simulink model "plant_block_swing"  (R2013a)
settings: Solver=ode1  StartTime=0.0  StopTime=120  RelTol=1e-3
undefined symbols (not defined in the file or in its folder): magnitude
libraries: simulink x2
settings Model: SimulationMode=external  ExtModeTrigDuration=50000  Creator=Dro  LastModifiedBy=s4358046
settings DataIOCC: LimitDataPoints=off  SignalLoggingSaveFormat=ModelDataLogs  SignalLoggingName=sigsOut
settings OptimizationCC: ExpressionDepthLimit=2147483647  InitFltsAndDblsToZero=on
settings DebuggingCC: SaveWithParameterizedLinksMsg=none  SignalResolutionControl=TryResolveAllWithWarning  SolverPrmCheckMsg=none  MultiTaskDSMMsg=warning  MultiTaskCondExecSysMsg=none  FcnCallInpInsideContextMsg=UseLocalSettings  StrictBusMsg=None
settings RTWCC: SystemTargetFile=rtwin.tlc  TemplateMakefile=rtwin.tmf  Description=Real-Time Windows Target  ProcessScript=rtwin_make_rtw_hook  IncludeERTFirstTime=on
settings RTWinTargetCC: TargetFcnLib=ansi_tfl_tmw.mat  TargetLibSuffix=_rtwin.lib  TargetPreCompLibLocation=C:\Program Files\MATLAB\R2013a\toolbox\rtw\targets\rtwin\lib\win64  CodeReplacementLibrary=ANSI_C  ModelReferenceCompliant=off  CompOptLevelCompliant=off  RTWinDir=C:/PROGRA~1/MATLAB/R2013a/toolbox/rtw/targets/rtwin  TargetArch=win64

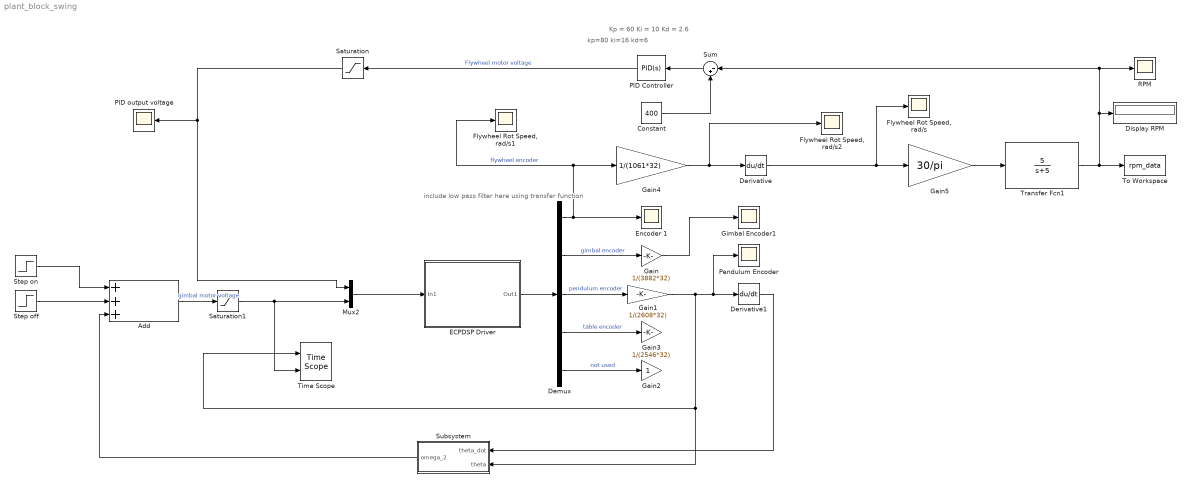
== system plant_block_swing ==
  note: Kp = 60
      | Ki = 10
      | Kd = 2.6
  note: include low pass filter here
      | using transfer function
  note: kp=80
      | ki=16
      | kd=6
  Add : Sum  Inputs=+++
  Constant : Constant  Value=400
  Demux : Demux  Outputs=5
  Derivative : Derivative
  Derivative1 : Derivative
  Display RPM : Display
  ECPDSP Driver : Subsystem  mask{BaseAddr='0xC000', STime=0.008, TimeOutPer=500, HWAccess=on}
      mask prompts: BaseAddr "Base I/O Address"; STime "Sample Time (Sec)"; TimeOutPer "Timeout Period (500 ~ 2000)"; HWAccess "Hardware Access"
      mask Display: color('black');disp('ECPDSP Driver\n upto\n 4 Encs(ADC Channels)\n and 2 Dacs')
  Encoder 1 : Scope
      settings: YMin=1.5e+06  YMax=8.5e+06  SaveName=ScopeData3
  "Flywheel Rot Speed, rad/s" : Scope
  "Flywheel Rot Speed, rad/s1" : Scope
      settings: SaveName=ScopeData2
  "Flywheel Rot Speed, rad/s2" : Scope
      settings: SaveName=ScopeData4
  Gain : Gain  Gain=1/(3882*32)
  Gain1 : Gain  Gain=1/(2608*32)
  Gain2 : Gain
  Gain3 : Gain  Gain=1/(2546*32)
  Gain4 : Gain  Gain=1/(1061*32)
  Gain5 : Gain  Gain=30/pi
  Gimbal Encoder1 : Scope
      settings: YMin=-0.25  YMax=3.25  SaveName=ScopeData9
  Mux2 : Mux  Inputs=2
  PID Controller : simulink/Continuous/PID Controller  Controller=PID  TimeDomain=Continuous-time  SampleTime=1  IntegratorMethod=Forward Euler  FilterMethod=Forward Euler  Form=Parallel  P=60  I=10  D=2.6  N=100  InitialConditionSource=internal  InitialConditionForIntegrator=0  InitialConditionForFilter=0  ExternalReset=none  LimitOutput=off  UpperSaturationLimit=inf  LowerSaturationLimit=-inf  LinearizeAsGain=on  AntiWindupMode=none  Kb=1  TrackingMode=off  Kt=1  PParamMin=[]  PParamMax=[]  IParamMin=[]  IParamMax=[]  DParamMin=[]  DParamMax=[]  NParamMin=[]  NParamMax=[]  KbParamMin=[]  KbParamMax=[]  KtParamMin=[]  KtParamMax=[]  POutMin=[]  POutMax=[]  IOutMin=[]  IOutMax=[]  DOutMin=[]  DOutMax=[]  NOutMin=[]  NOutMax=[]  KbOutMin=[]  KbOutMax=[]  KtOutMin=[]  KtOutMax=[]  IntegratorOutMin=[]  IntegratorOutMax=[]  FilterOutMin=[]  FilterOutMax=[]  SumOutMin=[]  SumOutMax=[]  SumI1OutMin=[]  SumI1OutMax=[]  SumI2OutMin=[]  SumI2OutMax=[]  SumI3OutMin=[]  SumI3OutMax=[]  SumDOutMin=[]  SumDOutMax=[]  SaturationOutMin=[]  SaturationOutMax=[]  IntegratorContinuousStateAttributes=''  IntegratorStateMustResolveToSignalObject=off  IntegratorRTWStateStorageClass=Auto  FilterContinuousStateAttributes=''  FilterStateMustResolveToSignalObject=off  FilterRTWStateStorageClass=Auto
  PID output voltage : Scope
      settings: YMin=400  YMax=421  SaveName=ScopeData6
  Pendulum Encoder : Scope
      settings: YMin=-0.25  YMax=3.25  SaveName=ScopeData5
  RPM : Scope
      settings: YMin=400  YMax=421
  Saturation : Saturate  UpperLimit=32000  LowerLimit=-32000
  Saturation1 : Saturate  UpperLimit=22000  LowerLimit=-22000
  Step off : Step  Time=30.15  After=-14000  SampleTime=0
  Step on : Step  Time=30  After=14000  SampleTime=0
  Subsystem : Subsystem
  Sum : Sum  Inputs=|-+
  Time Scope : TimeScope  NumInputPorts=2  DefaultConfigurationName=spbscopes.TimeScopeBlockCfg
      settings: CopyFcn=scopeextensions.ScopeBlock.callback(gcbh, 'onBlockCopy', gcbh);  DeleteFcn=scopeextensions.ScopeBlock.callback(gcbh, 'onBlockDelete');  PreSaveFcn=scopeextensions.ScopeBlock.callback(gcbh, 'onModelSave');  NameChangeFcn=scopeextensions.ScopeBlock.callback(gcbh, 'onBlockRename');  CloseFcn=scopeextensions.ScopeBlock.callback(gcbh, 'onBlockClose');  PreDeleteFcn=scopeextensions.ScopeBlock.callback(gcbh, 'onBlockPreDelete');
  To Workspace : ToWorkspace  VariableName=rpm_data  SampleTime=-1  SaveFormat=Timeseries
  Transfer Fcn1 : TransferFcn  Numerator=[5]  Denominator=[1 5]
  wires:
  ECPDSP Driver/1(Out1) -> Demux/1
  Demux/1 -> Encoder 1/1, Gain4/1, "Flywheel Rot Speed, rad/s1"/1  "flywheel encoder"
  PID Controller/1 -> Saturation/1  "Flywheel motor voltage"
  Demux/2 -> Gain/1  "gimbal encoder"
  Demux/3 -> Gain1/1  "pendulum encoder"
  Demux/4 -> Gain3/1  "table encoder"
  Demux/5 -> Gain2/1  "not used"
  Gain4/1 -> "Flywheel Rot Speed, rad/s2"/1, Derivative/1
  Constant/1 -> Sum/2
  Sum/1 -> PID Controller/1
  Saturation/1 -> PID output voltage/1, Mux2/1
  Derivative/1 -> Gain5/1, "Flywheel Rot Speed, rad/s"/1
  Gain5/1 -> Transfer Fcn1/1
  Step off/1 -> Add/2
  Step on/1 -> Add/1
  Add/1 -> Saturation1/1  "gimbal motor voltage"
  Derivative1/1 -> Subsystem/1(theta_dot)
  Subsystem/1(omega_2) -> Add/3
  Saturation1/1 -> Mux2/2, Time Scope/2
  Mux2/1 -> ECPDSP Driver/1(In1)
  Gain/1 -> Gimbal Encoder1/1
  Transfer Fcn1/1 -> To Workspace/1, Display RPM/1, RPM/1, Sum/1
  Gain1/1 -> Time Scope/1, Subsystem/2(theta), Pendulum Encoder/1, Derivative1/1

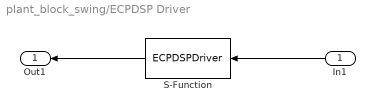
== system plant_block_swing/ECPDSP Driver ==
  In1 : Inport
  S-Function : S-Function  FunctionName=ECPDSPDriver  Parameters=BaseAddr,STime,TimeOutPer,HWAccess  EnableBusSupport=off
  Out1 : Outport
  wires:
  In1/1 -> S-Function/1
  S-Function/1 -> Out1/1

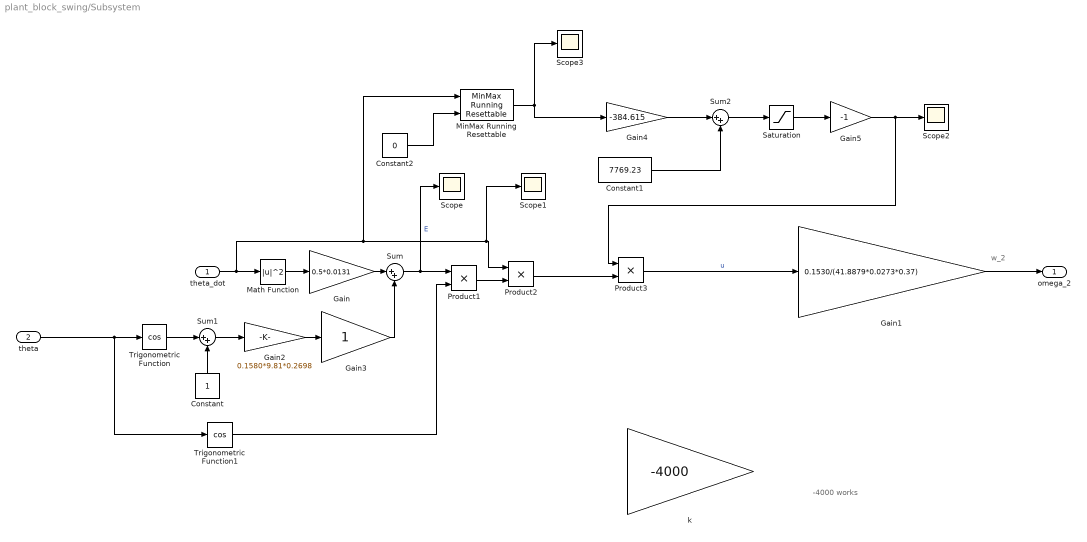
== system plant_block_swing/Subsystem ==
  note: -4000 works
  note: w_2
  theta_dot : Inport
  theta : Inport  Port=2
  Constant : Constant
  Constant1 : Constant  Value=7769.23
  Constant2 : Constant  Value=0
  Gain : Gain  Gain=0.5*0.0131
  Gain1 : Gain  Gain=0.1530/(41.8879*0.0273*0.37)
  Gain2 : Gain  Gain=0.1580*9.81*0.2698
  Gain3 : Gain
  Gain4 : Gain  Gain=-384.615
  Gain5 : Gain  Gain=-1
  Math Function : Math  Operator=magnitude^2  SaturateOnIntegerOverflow=on
  MinMax Running Resettable : simulink/Math Operations/MinMax Running Resettable  Function=max  vinit=0.0
  Product1 : Product
  Product2 : Product
  Product3 : Product
  Saturation : Saturate  UpperLimit=7000  LowerLimit=2000
  Scope{,1..3} (4 alike) : Scope
      Scope settings: SaveName=ScopeData7
      Scope1 settings: SaveName=ScopeData8
      Scope2 settings: SaveName=ScopeData10
      Scope3 settings: SaveName=ScopeData11
  Sum : Sum  Inputs=|++
  Sum1 : Sum  Inputs=|++
  Sum2 : Sum  Inputs=|++
  Trigonometric Function : Trigonometry  Operator=cos
  Trigonometric Function1 : Trigonometry  Operator=cos
  k : Gain  Gain=-4000
  omega_2 : Outport
  wires:
  theta_dot/1 -> MinMax Running Resettable/1, Scope1/1, Product2/1, Math Function/1
  Math Function/1 -> Gain/1
  Gain/1 -> Sum/1
  Product3/1 -> Gain1/1  "u"
  Gain1/1 -> omega_2/1
  Trigonometric Function/1 -> Sum1/1
  Constant/1 -> Sum1/2
  Sum1/1 -> Gain2/1
  Gain2/1 -> Gain3/1
  Sum/1 -> Product1/1, Scope/1  "E"
  Trigonometric Function1/1 -> Product1/2
  Product1/1 -> Product2/2
  Product2/1 -> Product3/2
  theta/1 -> Trigonometric Function1/1, Trigonometric Function/1
  Gain3/1 -> Sum/2
  MinMax Running Resettable/1 -> Gain4/1, Scope3/1
  Gain4/1 -> Sum2/1
  Constant1/1 -> Sum2/2
  Sum2/1 -> Saturation/1
  Saturation/1 -> Gain5/1
  Gain5/1 -> Product3/1, Scope2/1
  Constant2/1 -> MinMax Running Resettable/2
